simulink model "labs10"  (R2022b)
settings: Solver=VariableStepAuto  StartTime=0.0  StopTime=30  RelTol=1e-3
undefined symbols (not defined in the file or in its folder): K, Tm, Tt1, Tt2, Tt3
settings Model: Creator=micha  LastModifiedBy=mateu

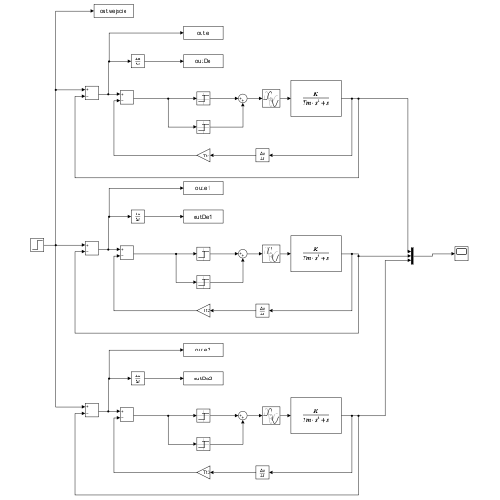
[thumbnail: Simulink's stored preview of the top-level diagram]
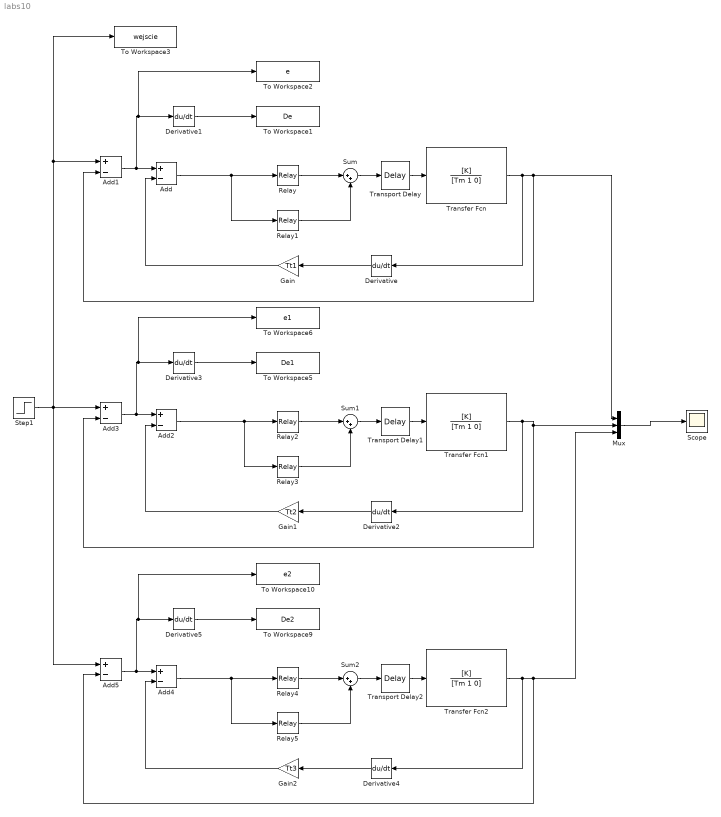
== system labs10 ==
  Add{,1..5} (6 alike) : Sum  Inputs=+-
  Derivative{,1..5} (6 alike) : Derivative
  Gain : Gain  Gain=Tt1
  Gain1 : Gain  Gain=Tt2
  Gain2 : Gain  Gain=Tt3
  Mux : Mux  Inputs=3
  Relay : Relay  OnSwitchValue=0.073  OffSwitchValue=0.05  OnOutputValue=3
  Relay1 : Relay  OnSwitchValue=-0.05  OffSwitchValue=-0.073  OnOutputValue=0  OffOutputValue=-3
  Relay2 : Relay  OnSwitchValue=0.073  OffSwitchValue=0.05  OnOutputValue=3
  Relay3 : Relay  OnSwitchValue=-0.05  OffSwitchValue=-0.073  OnOutputValue=0  OffOutputValue=-3
  Relay4 : Relay  OnSwitchValue=0.073  OffSwitchValue=0.05  OnOutputValue=3
  Relay5 : Relay  OnSwitchValue=-0.05  OffSwitchValue=-0.073  OnOutputValue=0  OffOutputValue=-3
  Scope : Scope
  Step1 : Step  Time=0  SampleTime=0.01
  Sum : Sum  Inputs=|++
  Sum1 : Sum  Inputs=|++
  Sum2 : Sum  Inputs=|++
  To Workspace1 : ToWorkspace  VariableName=De  SampleTime=-1
  To Workspace10 : ToWorkspace  VariableName=e2  SampleTime=-1
  To Workspace2 : ToWorkspace  VariableName=e  SampleTime=-1
  To Workspace3 : ToWorkspace  VariableName=wejscie  SampleTime=-1
  To Workspace5 : ToWorkspace  VariableName=De1  SampleTime=-1
  To Workspace6 : ToWorkspace  VariableName=e1  SampleTime=-1
  To Workspace9 : ToWorkspace  VariableName=De2  SampleTime=-1
  Transfer Fcn : TransferFcn  Numerator=[K]  Denominator=[Tm 1 0]
  Transfer Fcn1 : TransferFcn  Numerator=[K]  Denominator=[Tm 1 0]
  Transfer Fcn2 : TransferFcn  Numerator=[K]  Denominator=[Tm 1 0]
  Transport Delay : TransportDelay  DelayTime=0.11
  Transport Delay1 : TransportDelay  DelayTime=0.11
  Transport Delay2 : TransportDelay  DelayTime=0.11
  wires:
  Gain/1 -> Add/2
  Add/1 -> Relay1/1, Relay/1
  Derivative/1 -> Gain/1
  Derivative1/1 -> To Workspace1/1
  Sum/1 -> Transport Delay/1
  Transfer Fcn/1 -> Mux/1, Add1/2, Derivative/1
  Add1/1 -> To Workspace2/1, Derivative1/1, Add/1
  Relay1/1 -> Sum/2
  Transport Delay/1 -> Transfer Fcn/1
  Relay/1 -> Sum/1
  Gain1/1 -> Add2/2
  Add2/1 -> Relay3/1, Relay2/1
  Derivative2/1 -> Gain1/1
  Derivative3/1 -> To Workspace5/1
  Sum1/1 -> Transport Delay1/1
  Transfer Fcn1/1 -> Mux/2, Add3/2, Derivative2/1
  Step1/1 -> To Workspace3/1, Add1/1, Add5/1, Add3/1
  Add3/1 -> To Workspace6/1, Derivative3/1, Add2/1
  Transport Delay1/1 -> Transfer Fcn1/1
  Gain2/1 -> Add4/2
  Add4/1 -> Relay5/1, Relay4/1
  Derivative4/1 -> Gain2/1
  Derivative5/1 -> To Workspace9/1
  Sum2/1 -> Transport Delay2/1
  Transfer Fcn2/1 -> Mux/3, Add5/2, Derivative4/1
  Add5/1 -> To Workspace10/1, Derivative5/1, Add4/1
  Relay5/1 -> Sum2/2
  Transport Delay2/1 -> Transfer Fcn2/1
  Relay4/1 -> Sum2/1
  Mux/1 -> Scope/1
  Relay3/1 -> Sum1/2
  Relay2/1 -> Sum1/1
